simulink model "GCU_CAN_debug"  (R2018a)
settings: Solver=FixedStepAuto  StartTime=0.0  StopTime=10.0  FixedStep=0.01  RelTol=1e-3
settings Model: Creator=SIMONE  LastModifiedBy=SIMONE
settings SFSimCC: SimCustomHeaderCode=#define A 1

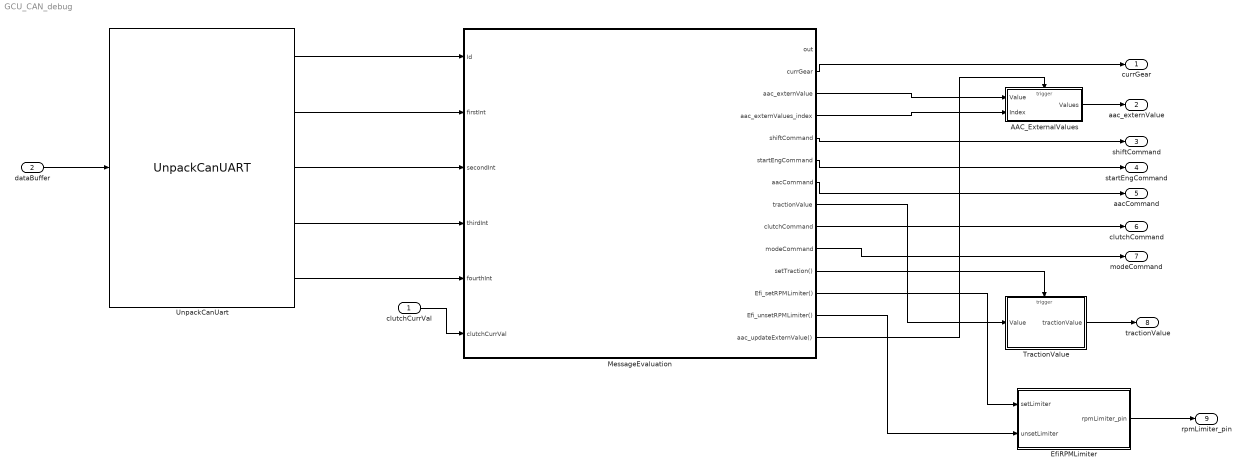
== system GCU_CAN_debug ==
  clutchCurrVal : Inport
  dataBuffer : Inport  Port=2
  AAC_ExternalValues : Subsystem  TreatAsAtomicUnit=on
  EfiRPMLimiter : Subsystem
  MessageEvaluation : Stateflow chart  TreatAsAtomicUnit=on  SystemSampleTime=0.01
  TractionValue : Subsystem  TreatAsAtomicUnit=on
  UnpackCanUart : S-Function  FunctionName=UnpackCanUART  SFunctionDeploymentMode=off  EnableBusSupport=off
  currGear : Outport
  aac_externValue : Outport  Port=2
  shiftCommand : Outport  Port=3
  startEngCommand : Outport  Port=4
  aacCommand : Outport  Port=5
  clutchCommand : Outport  Port=6
  modeCommand : Outport  Port=7
  tractionValue : Outport  Port=8
  rpmLimiter_pin : Outport  Port=9
  wires:
  MessageEvaluation/6(startEngCommand) -> startEngCommand/1
  EfiRPMLimiter/1(rpmLimiter_pin) -> rpmLimiter_pin/1
  UnpackCanUart/2 -> MessageEvaluation/2(firstInt)
  TractionValue/1(tractionValue) -> tractionValue/1
  UnpackCanUart/4 -> MessageEvaluation/4(thirdInt)
  MessageEvaluation/14(aac_updateExternValue()) -> AAC_ExternalValues/Trigger
  UnpackCanUart/3 -> MessageEvaluation/3(secondInt)
  MessageEvaluation/10(modeCommand) -> modeCommand/1
  MessageEvaluation/2(currGear) -> currGear/1
  clutchCurrVal/1 -> MessageEvaluation/6(clutchCurrVal)
  UnpackCanUart/5 -> MessageEvaluation/5(fourthInt)
  MessageEvaluation/3(aac_externValue) -> AAC_ExternalValues/1(Value)
  MessageEvaluation/7(aacCommand) -> aacCommand/1
  UnpackCanUart/1 -> MessageEvaluation/1(Id)
  MessageEvaluation/5(shiftCommand) -> shiftCommand/1
  MessageEvaluation/8(tractionValue) -> TractionValue/1(Value)
  AAC_ExternalValues/1(Values) -> aac_externValue/1
  dataBuffer/1 -> UnpackCanUart/1
  MessageEvaluation/4(aac_externValues_index) -> AAC_ExternalValues/2(Index)
  MessageEvaluation/13(Efi_unsetRPMLimiter()) -> EfiRPMLimiter/2(unsetLimiter)
  MessageEvaluation/9(clutchCommand) -> clutchCommand/1
  MessageEvaluation/11(setTraction()) -> TractionValue/Trigger
  MessageEvaluation/12(Efi_setRPMLimiter()) -> EfiRPMLimiter/1(setLimiter)

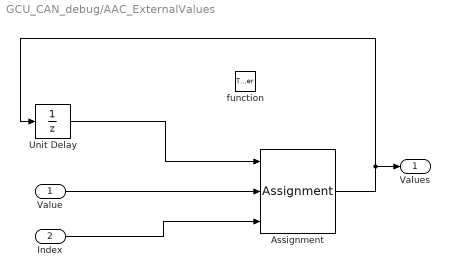
== system GCU_CAN_debug/AAC_ExternalValues ==
  Value : Inport
  Index : Inport  Port=2
  function : TriggerPort  TriggerType=function-call  VariantControl=Variant
  Assignment : Assignment  IndexMode=Zero-based  DiagnosticForDimensions=Warning  IndexOptions=Index vector (port)  Indices=1  OutputSizes=1
  Unit Delay : UnitDelay  InitialCondition=[0,0,0]  SampleTime=-1
  Values : Outport
  wires:
  Assignment/1 -> Unit Delay/1, Values/1
  Unit Delay/1 -> Assignment/1
  Value/1 -> Assignment/2
  Index/1 -> Assignment/3

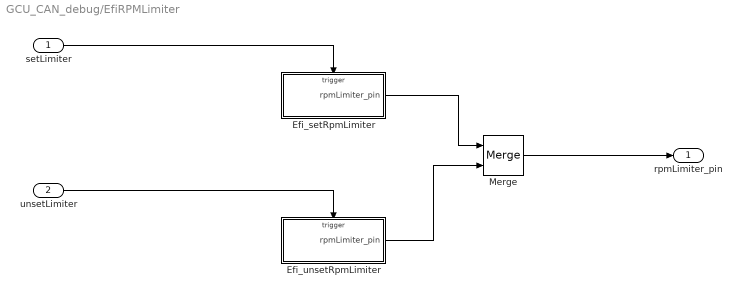
== system GCU_CAN_debug/EfiRPMLimiter ==
  setLimiter : Inport
  unsetLimiter : Inport  Port=2
  Efi_setRpmLimiter : Subsystem  TreatAsAtomicUnit=on
  Efi_unsetRpmLimiter : Subsystem  TreatAsAtomicUnit=on
  Merge : Merge
  rpmLimiter_pin : Outport
  wires:
  setLimiter/1 -> Efi_setRpmLimiter/Trigger
  unsetLimiter/1 -> Efi_unsetRpmLimiter/Trigger
  Efi_unsetRpmLimiter/1(rpmLimiter_pin) -> Merge/2
  Efi_setRpmLimiter/1(rpmLimiter_pin) -> Merge/1
  Merge/1 -> rpmLimiter_pin/1

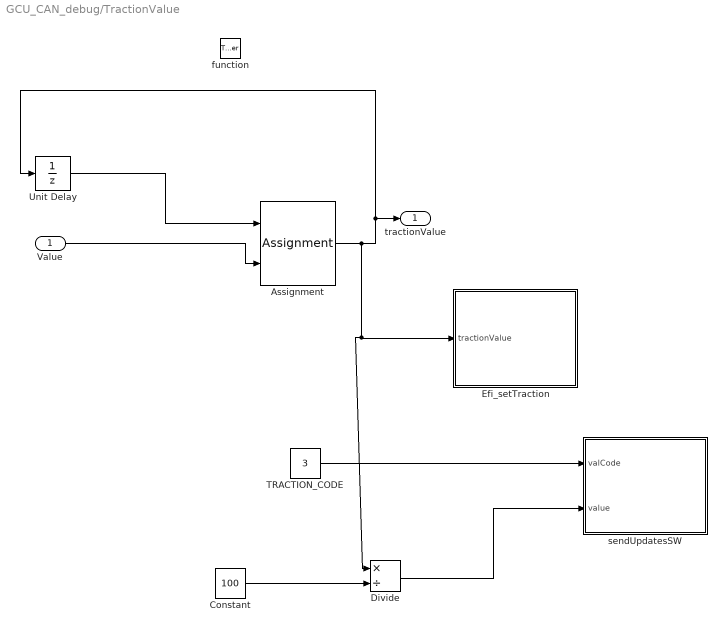
== system GCU_CAN_debug/TractionValue ==
  Value : Inport
  function : TriggerPort  TriggerType=function-call  VariantControl=Variant
  Assignment : Assignment  IndexMode=Zero-based  DiagnosticForDimensions=Warning  IndexOptions=Index vector (dialog)  Indices=0  OutputSizes=1
  Constant : Constant  Value=100  OutDataTypeStr=uint16
  Divide : Product  Inputs=*/
  Efi_setTraction : Subsystem
  TRACTION_CODE : Constant  Value=3  OutDataTypeStr=uint16
  Unit Delay : UnitDelay  SampleTime=-1
  sendUpdatesSW : Subsystem
  tractionValue : Outport
  wires:
  Value/1 -> Assignment/2
  Assignment/1 -> Divide/1, Efi_setTraction/1(tractionValue), Unit Delay/1, tractionValue/1
  Unit Delay/1 -> Assignment/1
  TRACTION_CODE/1 -> sendUpdatesSW/1(valCode)
  Constant/1 -> Divide/2
  Divide/1 -> sendUpdatesSW/2(value)

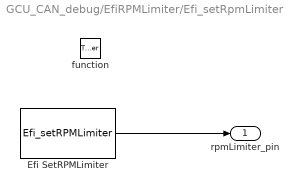
== system GCU_CAN_debug/EfiRPMLimiter/Efi_setRpmLimiter ==
  function : TriggerPort  TriggerType=function-call  VariantControl=Variant
  Efi SetRPMLimiter : S-Function  FunctionName=Efi_setRPMLimiter  SFunctionDeploymentMode=off  EnableBusSupport=off
  rpmLimiter_pin : Outport
  wires:
  Efi SetRPMLimiter/1 -> rpmLimiter_pin/1

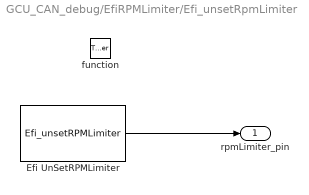
== system GCU_CAN_debug/EfiRPMLimiter/Efi_unsetRpmLimiter ==
  function : TriggerPort  TriggerType=function-call  VariantControl=Variant
  Efi UnSetRPMLimiter : S-Function  FunctionName=Efi_unsetRPMLimiter  SFunctionDeploymentMode=off  EnableBusSupport=off
  rpmLimiter_pin : Outport
  wires:
  Efi UnSetRPMLimiter/1 -> rpmLimiter_pin/1

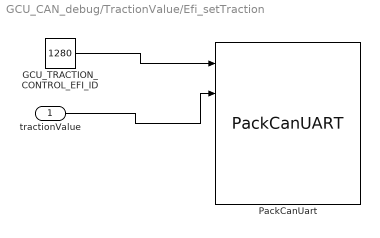
== system GCU_CAN_debug/TractionValue/Efi_setTraction ==
  tractionValue : Inport  OutDataTypeStr=uint16  PortDimensions=1
  GCU_TRACTION_CONTROL_EFI_ID : Constant  Value=1280  OutDataTypeStr=uint16
  PackCanUart : S-Function  FunctionName=PackCanUART  SFunctionDeploymentMode=off  EnableBusSupport=off
  wires:
  GCU_TRACTION_CONTROL_EFI_ID/1 -> PackCanUart/1
  tractionValue/1 -> PackCanUart/2

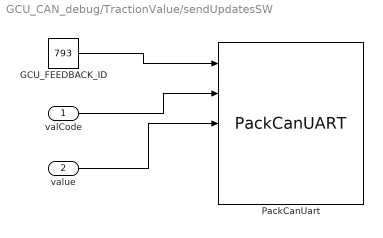
== system GCU_CAN_debug/TractionValue/sendUpdatesSW ==
  valCode : Inport  OutDataTypeStr=uint16  PortDimensions=1
  value : Inport  Port=2  OutDataTypeStr=uint16  PortDimensions=1
  GCU_FEEDBACK_ID : Constant  Value=793  OutDataTypeStr=uint16
  PackCanUart : S-Function  FunctionName=PackCanUART  SFunctionDeploymentMode=off  EnableBusSupport=off
  wires:
  GCU_FEEDBACK_ID/1 -> PackCanUart/1
  value/1 -> PackCanUart/3
  valCode/1 -> PackCanUart/2

== stateflow chart GCU_CAN_debug/MessageEvaluation ==
  state GEAR_RPM_UPDATE
    entry:
    currGear = firstInt;
    aac_externValues_index = uint16(aac_values.RPM);
    aac_externValue = secondInt;
    send(aac_updateExternValue);
  state IDLE
  state sendStartEngCommand [function]
    (default) -> (junction 280)
    (junction 280) -> (junction 281) [order 1] : [startEngCommand >= 255]
    (junction 280) -> (junction 282) [order 2] : {startEngCommand = startEngCommand + 1;}
    (junction 281) -> (junction 283) : {startEngCommand = 0}
  state START_ENGINE
    entry:
    sendStartEngCommand();
  state SW_GEARSHIFT
    state SetLimiter
      entry:
      send(Efi_setRPMLimiter);
    state UnsetLimiter
      entry:
      send(Efi_unsetRPMLimiter);
    state START_SHIFT
      entry:
      sendShiftCommand(firstInt);
    (default) -> (junction 113)
    (junction 113) -> SetLimiter [order 1] : [firstInt== RPM_LIMITER_ON]
    (junction 113) -> (junction 126) [order 2]
    (junction 126) -> UnsetLimiter [order 1] : [firstInt== RPM_LIMITER_OFF]
    (junction 126) -> START_SHIFT [order 2]
  state sendShiftCommand(com) [function]
    (default) -> (junction 211)
    (junction 211) -> (junction 212) [order 1] : [shiftCommand[0] >= 255]
    (junction 211) -> (junction 214) [order 2] : {shiftCommand[0] = shiftCommand[0] + 1}
    (junction 212) -> (junction 215) : {shiftCommand[0] = 0}
    (junction 214) -> (junction 215)
    (junction 215) -> (junction 216) : {shiftCommand[1] = com}
    (junction 216) -> (junction 224) [order 1] : [clutchCurrVal ~= 100]
    (junction 216) -> (junction 229) [order 2]
    (junction 224) -> (junction 226)
    (junction 226) -> (junction 305) [order 1] : [(com == GEAR_COMMAND_NEUTRAL_UP) || (com == GEAR_COMMAND_NEUTRAL_DOWN) ||  (com == GEAR_COMMAND_DOWN) ]
    (junction 226) -> (junction 307) [order 2]
    (junction 305) -> (junction 309) : {sendAacCommand(STOP_COM)}
  state sendClutchCommand(com) [function]
    (default) -> (junction 187)
    (junction 187) -> (junction 188) [order 1] : [clutchCommand[0] >= 255]
    (junction 187) -> (junction 190) [order 2] : {clutchCommand[0] = clutchCommand[0] + 1}
    (junction 188) -> (junction 191) : {clutchCommand[0] = 0}
    (junction 190) -> (junction 191)
    (junction 191) -> (junction 192) : {clutchCommand[1] = com}
  state WHEEL_SPEED_UPDATE
    entry:
    aac_externValues_index = uint16(aac_values.WHEEL_SPEED)
    aac_externValue = firstInt/10;
    send(aac_updateExternValue);
  state SET_CLUTCH
    entry:
    clutchSetVal = firstInt>>8;
    (default) -> (junction 263)
    (junction 263) -> (junction 267) [order 1] : [clutchSetVal > AAC_CLUTCH_NOISE_LEVEL]
    (junction 263) -> (junction 271) [order 2]
    (junction 267) -> (junction 269) : {sendAacCommand(STOP_COM);}
    (junction 271) -> (junction 269)
    (junction 269) -> (junction 274) : {sendClutchCommand(clutchSetVal);}
  state sendAacCommand(com) [function]
    (default) -> (junction 164)
    (junction 164) -> (junction 167) [order 1] : [aacCommand[0] >= 255]
    (junction 164) -> (junction 171) [order 2] : {aacCommand[0] = aacCommand[0] + 1}
    (junction 167) -> (junction 169) : {aacCommand[0] = 0}
    (junction 169) -> (junction 173)
    (junction 171) -> (junction 173)
    (junction 173) -> (junction 176) : {aacCommand[1] = com}
  state AAC_COM
    (default) -> (junction 253)
    (junction 253) -> (junction 255) : {sendAacCommand(firstInt);}
    (junction 255) -> (junction 257) [order 1] : [aacCommand[1] == STOP_COM]
    (junction 255) -> (junction 259) [order 2]
    (junction 257) -> (junction 261) : {sendClutchCommand(uint8(0))}
  state sendModeCommand(com) [function]
    (default) -> (junction 324)
    (junction 324) -> (junction 325) [order 1] : [modeCommand[0] >= 255]
    (junction 324) -> (junction 327) [order 2] : {modeCommand[0] = modeCommand[0] + 1}
    (junction 325) -> (junction 328) : {modeCommand[0] = 0}
    (junction 327) -> (junction 328)
    (junction 328) -> (junction 329) : {modeCommand[1] = com}
  state SET_TRACTION
    entry:
    tractionValue = uint16(firstInt) * 100;
    send(setTraction);
  state SW_CHANGE_MODE
    entry:
    sendModeCommand(firstInt);
  note: Indirizzo da decidere
  (junction 72) -> (junction 44)
  (default) -> IDLE
  GEAR_RPM_UPDATE -> (junction 72)
  (junction 75) -> (junction 72)
  IDLE -> (junction 44)
  (junction 44) -> GEAR_RPM_UPDATE [order 1] : [Id == EFI_GEAR_RPM_TPS_APPS_ID]
  (junction 44) -> (junction 51) [order 2]
  (junction 311) -> IDLE [order 2]
  START_ENGINE -> (junction 75)
  (junction 76) -> (junction 75)
  (junction 51) -> START_ENGINE [order 1] : [Id == SW_FIRE_GCU_ID]
  (junction 51) -> (junction 57) [order 2]
  (junction 57) -> SW_GEARSHIFT [order 1] : [Id == SW_GEARSHIFT_ID]
  SW_GEARSHIFT -> (junction 76)
  (junction 57) -> (junction 62) [order 2]
  (junction 77) -> (junction 76)
  WHEEL_SPEED_UPDATE -> (junction 77)
  (junction 78) -> (junction 77)
  (junction 62) -> WHEEL_SPEED_UPDATE [order 1] : [Id == EFI_TRACTION_CONTROL_ID]
  (junction 62) -> (junction 67) [order 2]
  SET_CLUTCH -> (junction 78)
  (junction 67) -> SET_CLUTCH [order 1] : [Id==SW_CLUTCH_TARGET_GCU_ID]
  (junction 67) -> (junction 145) [order 2]
  (junction 149) -> (junction 78)
  (junction 145) -> AAC_COM [order 1] : [Id == SW_ACCELERATION_GCU_ID]
  AAC_COM -> (junction 149)
  (junction 145) -> (junction 153) [order 2]
  (junction 157) -> (junction 149)
  (junction 153) -> SET_TRACTION [order 1] : [Id == SW_TRACTION_CONTROL_GCU_ID]
  SET_TRACTION -> (junction 157)
  (junction 153) -> (junction 311) [order 2]
  (junction 317) -> (junction 157)
  (junction 311) -> SW_CHANGE_MODE [order 1] : [Id == SW_MODE_ID]
  SW_CHANGE_MODE -> (junction 317)
  data: STOP_COM constant uint16 =uint16(0); RPM_LIMITER_ON constant uint16 =150; RPM_LIMITER_OFF constant uint16 =160; com function_input uint16 size=1; STOP_COM constant uint16 =uint16(0); GEAR_COMMAND_NEUTRAL_DOWN constant uint16 =uint16(100); GEAR_COMMAND_NEUTRAL_UP constant uint16 =uint16(50); GEAR_COMMAND_DOWN constant uint16 =uint16(200); com function_input uint16 size=1; STOP_COM constant uint16 =uint16(0); AAC_CLUTCH_NOISE_LEVEL constant uint8 =uint8(30); clutchSetVal local uint8 size=1; com function_input uint16 size=1; STOP_COM constant uint16 =uint16(0); STOP_COM constant uint16 =uint16(0); com function_input uint16 size=1; Id input uint16 size=1; firstInt input uint16 size=1; secondInt input uint16 size=1; thirdInt input uint16 size=1; fourthInt input uint16 size=1; EFI_TRACTION_CONTROL_ID constant uint16 size=1 =uint16(774); SW_FIRE_GCU_ID constant uint16 size=1 =516; SW_CLUTCH_TARGET_GCU_ID constant uint16 size=1 =uint16(513); EFI_GEAR_RPM_TPS_APPS_ID constant uint16 size=1 =uint16(773); out output size=1 =0; currGear output uint16 size=1 [..uint16(5)] =uint16(0); aac_externValue output uint16 size=1 =uint16(0); aac_externValues_index output uint16 size=1 [..uint16(3)] =uint16(0); AAC_NUM_VALUES constant uint16 size=1 =3; shiftCommand output uint16 size=[1, 2] =[uint16(0), uint16(0)]; SW_ACCELERATION_GCU_ID constant uint16 size=1 =uint16(514); SW_TRACTION_CONTROL_GCU_ID constant uint16 size=1 =uint16(515); startEngCommand output uint8 size=1 =uint8(0); aacCommand output uint16 size=[1,2] =[uint16(0), uint16(0)]; tractionValue output uint16 size=1; clutchCommand output uint8 size=[1,2] =[uint8(0), uint8(0)]; clutchCurrVal input uint8 size=1; SW_MODE_ID constant uint16 size=1 =uint16(1000); modeCommand output uint16 size=[1,2] =[uint16(0), uint16(0)]; SW_GEARSHIFT_ID constant double size=1 =uint16(512)
  events: setTraction output FUNCTION_CALL_EVENT; Efi_setRPMLimiter output FUNCTION_CALL_EVENT; Efi_unsetRPMLimiter output FUNCTION_CALL_EVENT; aac_updateExternValue output FUNCTION_CALL_EVENT
